simulink model "EMB_simplified"  (R2013b)
settings: Solver=ode45  StartTime=0.0  StopTime=0.2  RelTol=1e-3
values from neighbouring files (symbols this model uses):
  d_rot = 0.1    [init_parameters.m]
  i = 113.1167    [init_parameters.m]
  K = 0.02    [init_parameters.m]
  K_I = 1000    [init_parameters.m]
  K_P = 10000    [init_parameters.m]
  L = 1e-3    (= 0.001)    [init_parameters.m]
  R = 0.3    [init_parameters.m]
  x0 = 0.05    [init_parameters.m]
settings Model: Creator=thomasst  LastModifiedBy=oej2si
settings DataIOCC: SignalLoggingSaveFormat=ModelDataLogs
settings DebuggingCC: UnderspecifiedInitializationDetection=Simplified  MergeDetectMultiDrivingBlocksExec=error  MultiTaskDSMMsg=warning  MultiTaskCondExecSysMsg=none  StrictBusMsg=None
settings RTWCC: IncludeERTFirstTime=on
settings GRTTargetCC: CodeReplacementLibrary=None  CPPClassGenCompliant=on

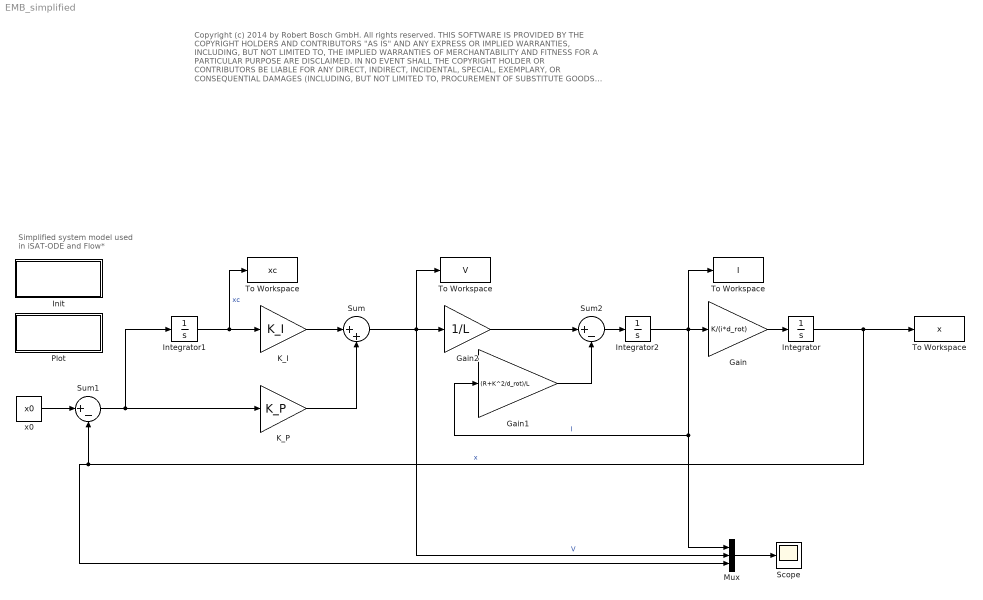
== system EMB_simplified ==
  note: Copyright (c) 2014 by Robert Bosch GmbH. All rights reserved.
      |
      | THIS SOFTWARE IS PROVIDED BY THE COPYRIGHT HOLDERS AND CONTRIBUTORS "AS IS"
      | AND ANY EXPRESS OR IMPLIED WARRANTIES, INCLUDING, BUT NOT LIMITED TO, THE IMPLIED
      | WARRANTIES OF MERCHANTABILITY AND FITNESS FOR A PARTICULAR PURPOSE ARE
      | DISCLAIMED. IN NO EVENT SHALL THE COPYRIGHT HOLDER OR CONTRIBUTORS BE LIABLE FOR
      | ANY DIRECT, INDIRECT, INCIDENTAL, SPECIAL, EXEMPLARY, OR CONSEQUENTIAL DAMAGES
      |  (INCLUDING, BUT NOT LIMITED TO, PROCUREMENT OF SUBSTITUTE GOODS OR SERVICES;
      | LOSS OF USE, DATA, OR PROFITS; OR BUSINESS INTERRUPTION) HOWEVER CAUSED AND
      | ON ANY THEORY OF LIABILITY, WHETHER IN CONTRACT, STRICT LIABILITY, OR TORT (INCLUDING
      | NEGLIGENCE OR OTHERWISE) ARISING IN ANY WAY OUT OF THE USE OF THIS SOFTWARE, EVEN
      | IF ADVISED OF THE POSSIBILITY OF SUCH DAMAGE.
      |
      | THE ENTIRE RISK AS TO THE QUALITY AND PERFORMANCE OF THE PROGRAM IS WITH YOU. SHOULD THE PROGRAM PROVE DEFECTIVE, YOU ASSUME THE COST OF ALL NECESSARY SERVICING, REPAIR OR CORRECTION.
      |
      | This is not a model of a Bosch product.
      | This model was originally released in the scope of the ARCH workshop (http://cps-vo.org/group/ARCH).
  note: Simplified system model used in iSAT-ODE and Flow*
  "  To Workspace " : ToWorkspace  VariableName=I  SampleTime=-1
  "  To Workspace  " : ToWorkspace  VariableName=xc  SampleTime=-1
  " To Workspace " : ToWorkspace  VariableName=V  SampleTime=-1
  Gain : Gain  Gain=K/(i*d_rot)
  Gain1 : Gain  Gain=(R+K^2/d_rot)/L
  Gain2 : Gain  Gain=1/L
  Init : Subsystem
      settings: OpenFcn=init_parameters
  Integrator : Integrator
  Integrator1 : Integrator
  Integrator2 : Integrator
  K_I : Gain  Gain=K_I
  K_P : Gain  Gain=K_P
  Mux : Mux  Inputs=3
  Plot : Subsystem
      settings: OpenFcn=plot_statevars
  Scope : Scope
      settings: TimeRange=0.16  YMin=0  YMax=900
  Sum : Sum  Inputs=|++
  Sum1 : Sum  Inputs=|+-
  Sum2 : Sum  Inputs=|+-
  To Workspace : ToWorkspace  VariableName=x  SampleTime=-1
  x0 : Constant  Value=x0
  wires:
  Gain/1 -> Integrator/1
  Integrator/1 -> To Workspace/1, Mux/3, Sum1/2  "x"
  x0/1 -> Sum1/1
  Sum1/1 -> K_P/1, Integrator1/1
  Integrator1/1 -> K_I/1, "  To Workspace  "/1  "xc"
  K_I/1 -> Sum/1
  K_P/1 -> Sum/2
  Sum/1 -> Mux/2, " To Workspace "/1, Gain2/1  "V"
  Integrator2/1 -> "  To Workspace "/1, Gain/1, Mux/1, Gain1/1  "I"
  Gain2/1 -> Sum2/1
  Sum2/1 -> Integrator2/1
  Gain1/1 -> Sum2/2
  Mux/1 -> Scope/1

== system EMB_simplified/Init ==

== system EMB_simplified/Plot ==
